simulink model "gm_robot_fis"  (R2023a)
settings: Solver=FixedStepDiscrete  StartTime=0.0  StopTime=10.0  RelTol=1e-3
model workspace (MAT data in the model file):
  x = 1
  y = [100 100 100 100 100 100 100 100 100 100 100 100 ... (256 elements, 256x1)]
libraries: hdlmdlgenlib x75
(part 2 of 3)

== system gm_robot_fis/MATLAB Function ==
  a : Inport  OutDataTypeStr=uint8  PortDimensions=1  SampleTime=0.2
  b : Inport  Port=2  OutDataTypeStr=uint8  PortDimensions=1  SampleTime=0.2
  c : Inport  Port=3  OutDataTypeStr=uint8  PortDimensions=1  SampleTime=0.2
  d : Inport  Port=4  OutDataTypeStr=uint8  PortDimensions=1  SampleTime=0.2
  e : Inport  Port=5  OutDataTypeStr=uint8  PortDimensions=1  SampleTime=0.2
  MATLAB Function : MATLAB Function  TreatAsAtomicUnit=on
  y : Outport  SampleTime=0.2
  wires:
  MATLAB Function/1(y) -> y/1
  a/1 -> MATLAB Function/1(a)
  b/1 -> MATLAB Function/2(b)
  c/1 -> MATLAB Function/3(c)
  d/1 -> MATLAB Function/4(d)
  e/1 -> MATLAB Function/5(e)

== system gm_robot_fis/MinMax Running Resettable ==
  note: Reset
  u : Inport  OutDataTypeStr=uint8  SampleTime=0.2
  R : Inport  Port=2  OutDataTypeStr=uint8  SampleTime=0.2
  Data Type Duplicate : DataTypeDuplicate  DisableCoverage=on  NumInputPorts=3
  MinMax : MinMax  DisableCoverage=on  Inputs=2  OutDataTypeStr=Inherit: Inherit via back propagation  ZeroCross=off
      settings: LockScale=on
  MinMax_out1 : hdlmdlgenlib/Buffer
  Subsystem : Subsystem
  Subsystem_out1 : hdlmdlgenlib/Buffer
  Subsystem_out2 : hdlmdlgenlib/Buffer
  y : Outport  SampleTime=0.2
  wires:
  MinMax_out1/1 -> Data Type Duplicate/1
  Subsystem_out1/1 -> y/1
  Subsystem_out2/1 -> Data Type Duplicate/2
  u/1 -> Data Type Duplicate/3, MinMax/1
  R/1 -> Subsystem/2(R1)
  MinMax/1 -> MinMax_out1/1, Subsystem/1(u1)
  Subsystem/1(y1) -> Subsystem_out1/1
  Subsystem/2(x) -> Subsystem_out2/1, MinMax/2

== system gm_robot_fis/MinMax Running Resettable1 ==
  note: Reset
  u : Inport  OutDataTypeStr=uint8  SampleTime=0.2
  R : Inport  Port=2  OutDataTypeStr=uint8  SampleTime=0.2
  Data Type Duplicate : DataTypeDuplicate  DisableCoverage=on  NumInputPorts=3
  MinMax : MinMax  DisableCoverage=on  Inputs=2  OutDataTypeStr=Inherit: Inherit via back propagation  ZeroCross=off
      settings: LockScale=on
  MinMax_out1 : hdlmdlgenlib/Buffer
  Subsystem : Subsystem
  Subsystem_out1 : hdlmdlgenlib/Buffer
  Subsystem_out2 : hdlmdlgenlib/Buffer
  y : Outport  SampleTime=0.2
  wires:
  MinMax_out1/1 -> Data Type Duplicate/1
  Subsystem_out1/1 -> y/1
  Subsystem_out2/1 -> Data Type Duplicate/2
  u/1 -> Data Type Duplicate/3, MinMax/1
  R/1 -> Subsystem/2(R1)
  MinMax/1 -> MinMax_out1/1, Subsystem/1(u1)
  Subsystem/1(y1) -> Subsystem_out1/1
  Subsystem/2(x) -> Subsystem_out2/1, MinMax/2

== system gm_robot_fis/MinMax Running Resettable10 ==
  note: Reset
  u : Inport  OutDataTypeStr=uint8  SampleTime=0.2
  R : Inport  Port=2  OutDataTypeStr=uint8  SampleTime=0.2
  Data Type Duplicate : DataTypeDuplicate  DisableCoverage=on  NumInputPorts=3
  MinMax : MinMax  DisableCoverage=on  Inputs=2  OutDataTypeStr=Inherit: Inherit via back propagation  ZeroCross=off
      settings: LockScale=on
  MinMax_out1 : hdlmdlgenlib/Buffer
  Subsystem : Subsystem
  Subsystem_out1 : hdlmdlgenlib/Buffer
  Subsystem_out2 : hdlmdlgenlib/Buffer
  y : Outport  SampleTime=0.2
  wires:
  MinMax_out1/1 -> Data Type Duplicate/1
  Subsystem_out1/1 -> y/1
  Subsystem_out2/1 -> Data Type Duplicate/2
  u/1 -> Data Type Duplicate/3, MinMax/1
  R/1 -> Subsystem/2(R1)
  MinMax/1 -> MinMax_out1/1, Subsystem/1(u1)
  Subsystem/1(y1) -> Subsystem_out1/1
  Subsystem/2(x) -> Subsystem_out2/1, MinMax/2

== system gm_robot_fis/MinMax Running Resettable11 ==
  note: Reset
  u : Inport  OutDataTypeStr=uint8  SampleTime=0.2
  R : Inport  Port=2  OutDataTypeStr=uint8  SampleTime=0.2
  Data Type Duplicate : DataTypeDuplicate  DisableCoverage=on  NumInputPorts=3
  MinMax : MinMax  DisableCoverage=on  Inputs=2  OutDataTypeStr=Inherit: Inherit via back propagation  ZeroCross=off
      settings: LockScale=on
  MinMax_out1 : hdlmdlgenlib/Buffer
  Subsystem : Subsystem
  Subsystem_out1 : hdlmdlgenlib/Buffer
  Subsystem_out2 : hdlmdlgenlib/Buffer
  y : Outport  SampleTime=0.2
  wires:
  MinMax_out1/1 -> Data Type Duplicate/1
  Subsystem_out1/1 -> y/1
  Subsystem_out2/1 -> Data Type Duplicate/2
  u/1 -> Data Type Duplicate/3, MinMax/1
  R/1 -> Subsystem/2(R1)
  MinMax/1 -> MinMax_out1/1, Subsystem/1(u1)
  Subsystem/1(y1) -> Subsystem_out1/1
  Subsystem/2(x) -> Subsystem_out2/1, MinMax/2

== system gm_robot_fis/MinMax Running Resettable12 ==
  note: Reset
  u : Inport  OutDataTypeStr=uint8  SampleTime=0.2
  R : Inport  Port=2  OutDataTypeStr=uint8  SampleTime=0.2
  Data Type Duplicate : DataTypeDuplicate  DisableCoverage=on  NumInputPorts=3
  MinMax : MinMax  DisableCoverage=on  Inputs=2  OutDataTypeStr=Inherit: Inherit via back propagation  ZeroCross=off
      settings: LockScale=on
  MinMax_out1 : hdlmdlgenlib/Buffer
  Subsystem : Subsystem
  Subsystem_out1 : hdlmdlgenlib/Buffer
  Subsystem_out2 : hdlmdlgenlib/Buffer
  y : Outport  SampleTime=0.2
  wires:
  MinMax_out1/1 -> Data Type Duplicate/1
  Subsystem_out1/1 -> y/1
  Subsystem_out2/1 -> Data Type Duplicate/2
  u/1 -> Data Type Duplicate/3, MinMax/1
  R/1 -> Subsystem/2(R1)
  MinMax/1 -> MinMax_out1/1, Subsystem/1(u1)
  Subsystem/1(y1) -> Subsystem_out1/1
  Subsystem/2(x) -> Subsystem_out2/1, MinMax/2

== system gm_robot_fis/MinMax Running Resettable13 ==
  note: Reset
  u : Inport  OutDataTypeStr=uint8  SampleTime=0.2
  R : Inport  Port=2  OutDataTypeStr=uint8  SampleTime=0.2
  Data Type Duplicate : DataTypeDuplicate  DisableCoverage=on  NumInputPorts=3
  MinMax : MinMax  DisableCoverage=on  Inputs=2  OutDataTypeStr=Inherit: Inherit via back propagation  ZeroCross=off
      settings: LockScale=on
  MinMax_out1 : hdlmdlgenlib/Buffer
  Subsystem : Subsystem
  Subsystem_out1 : hdlmdlgenlib/Buffer
  Subsystem_out2 : hdlmdlgenlib/Buffer
  y : Outport  SampleTime=0.2
  wires:
  MinMax_out1/1 -> Data Type Duplicate/1
  Subsystem_out1/1 -> y/1
  Subsystem_out2/1 -> Data Type Duplicate/2
  u/1 -> Data Type Duplicate/3, MinMax/1
  R/1 -> Subsystem/2(R1)
  MinMax/1 -> MinMax_out1/1, Subsystem/1(u1)
  Subsystem/1(y1) -> Subsystem_out1/1
  Subsystem/2(x) -> Subsystem_out2/1, MinMax/2

== system gm_robot_fis/MinMax Running Resettable14 ==
  note: Reset
  u : Inport  OutDataTypeStr=uint8  SampleTime=0.2
  R : Inport  Port=2  OutDataTypeStr=uint8  SampleTime=0.2
  Data Type Duplicate : DataTypeDuplicate  DisableCoverage=on  NumInputPorts=3
  MinMax : MinMax  DisableCoverage=on  Inputs=2  OutDataTypeStr=Inherit: Inherit via back propagation  ZeroCross=off
      settings: LockScale=on
  MinMax_out1 : hdlmdlgenlib/Buffer
  Subsystem : Subsystem
  Subsystem_out1 : hdlmdlgenlib/Buffer
  Subsystem_out2 : hdlmdlgenlib/Buffer
  y : Outport  SampleTime=0.2
  wires:
  MinMax_out1/1 -> Data Type Duplicate/1
  Subsystem_out1/1 -> y/1
  Subsystem_out2/1 -> Data Type Duplicate/2
  u/1 -> Data Type Duplicate/3, MinMax/1
  R/1 -> Subsystem/2(R1)
  MinMax/1 -> MinMax_out1/1, Subsystem/1(u1)
  Subsystem/1(y1) -> Subsystem_out1/1
  Subsystem/2(x) -> Subsystem_out2/1, MinMax/2

== system gm_robot_fis/MinMax Running Resettable15 ==
  note: Reset
  u : Inport  OutDataTypeStr=uint8  SampleTime=0.2
  R : Inport  Port=2  OutDataTypeStr=uint8  SampleTime=0.2
  Data Type Duplicate : DataTypeDuplicate  DisableCoverage=on  NumInputPorts=3
  MinMax : MinMax  DisableCoverage=on  Inputs=2  OutDataTypeStr=Inherit: Inherit via back propagation  ZeroCross=off
      settings: LockScale=on
  MinMax_out1 : hdlmdlgenlib/Buffer
  Subsystem : Subsystem
  Subsystem_out1 : hdlmdlgenlib/Buffer
  Subsystem_out2 : hdlmdlgenlib/Buffer
  y : Outport  SampleTime=0.2
  wires:
  MinMax_out1/1 -> Data Type Duplicate/1
  Subsystem_out1/1 -> y/1
  Subsystem_out2/1 -> Data Type Duplicate/2
  u/1 -> Data Type Duplicate/3, MinMax/1
  R/1 -> Subsystem/2(R1)
  MinMax/1 -> MinMax_out1/1, Subsystem/1(u1)
  Subsystem/1(y1) -> Subsystem_out1/1
  Subsystem/2(x) -> Subsystem_out2/1, MinMax/2

== system gm_robot_fis/MinMax Running Resettable16 ==
  note: Reset
  u : Inport  OutDataTypeStr=uint8  SampleTime=0.2
  R : Inport  Port=2  OutDataTypeStr=uint8  SampleTime=0.2
  Data Type Duplicate : DataTypeDuplicate  DisableCoverage=on  NumInputPorts=3
  MinMax : MinMax  DisableCoverage=on  Inputs=2  OutDataTypeStr=Inherit: Inherit via back propagation  ZeroCross=off
      settings: LockScale=on
  MinMax_out1 : hdlmdlgenlib/Buffer
  Subsystem : Subsystem
  Subsystem_out1 : hdlmdlgenlib/Buffer
  Subsystem_out2 : hdlmdlgenlib/Buffer
  y : Outport  SampleTime=0.2
  wires:
  MinMax_out1/1 -> Data Type Duplicate/1
  Subsystem_out1/1 -> y/1
  Subsystem_out2/1 -> Data Type Duplicate/2
  u/1 -> Data Type Duplicate/3, MinMax/1
  R/1 -> Subsystem/2(R1)
  MinMax/1 -> MinMax_out1/1, Subsystem/1(u1)
  Subsystem/1(y1) -> Subsystem_out1/1
  Subsystem/2(x) -> Subsystem_out2/1, MinMax/2

== system gm_robot_fis/MinMax Running Resettable17 ==
  note: Reset
  u : Inport  OutDataTypeStr=uint8  SampleTime=0.2
  R : Inport  Port=2  OutDataTypeStr=uint8  SampleTime=0.2
  Data Type Duplicate : DataTypeDuplicate  DisableCoverage=on  NumInputPorts=3
  MinMax : MinMax  DisableCoverage=on  Inputs=2  OutDataTypeStr=Inherit: Inherit via back propagation  ZeroCross=off
      settings: LockScale=on
  MinMax_out1 : hdlmdlgenlib/Buffer
  Subsystem : Subsystem
  Subsystem_out1 : hdlmdlgenlib/Buffer
  Subsystem_out2 : hdlmdlgenlib/Buffer
  y : Outport  SampleTime=0.2
  wires:
  MinMax_out1/1 -> Data Type Duplicate/1
  Subsystem_out1/1 -> y/1
  Subsystem_out2/1 -> Data Type Duplicate/2
  u/1 -> Data Type Duplicate/3, MinMax/1
  R/1 -> Subsystem/2(R1)
  MinMax/1 -> MinMax_out1/1, Subsystem/1(u1)
  Subsystem/1(y1) -> Subsystem_out1/1
  Subsystem/2(x) -> Subsystem_out2/1, MinMax/2

== system gm_robot_fis/MinMax Running Resettable18 ==
  note: Reset
  u : Inport  OutDataTypeStr=uint8  SampleTime=0.2
  R : Inport  Port=2  OutDataTypeStr=uint8  SampleTime=0.2
  Data Type Duplicate : DataTypeDuplicate  DisableCoverage=on  NumInputPorts=3
  MinMax : MinMax  DisableCoverage=on  Inputs=2  OutDataTypeStr=Inherit: Inherit via back propagation  ZeroCross=off
      settings: LockScale=on
  MinMax_out1 : hdlmdlgenlib/Buffer
  Subsystem : Subsystem
  Subsystem_out1 : hdlmdlgenlib/Buffer
  Subsystem_out2 : hdlmdlgenlib/Buffer
  y : Outport  SampleTime=0.2
  wires:
  MinMax_out1/1 -> Data Type Duplicate/1
  Subsystem_out1/1 -> y/1
  Subsystem_out2/1 -> Data Type Duplicate/2
  u/1 -> Data Type Duplicate/3, MinMax/1
  R/1 -> Subsystem/2(R1)
  MinMax/1 -> MinMax_out1/1, Subsystem/1(u1)
  Subsystem/1(y1) -> Subsystem_out1/1
  Subsystem/2(x) -> Subsystem_out2/1, MinMax/2

== system gm_robot_fis/MinMax Running Resettable19 ==
  note: Reset
  u : Inport  OutDataTypeStr=uint8  SampleTime=0.2
  R : Inport  Port=2  OutDataTypeStr=uint8  SampleTime=0.2
  Data Type Duplicate : DataTypeDuplicate  DisableCoverage=on  NumInputPorts=3
  MinMax : MinMax  DisableCoverage=on  Inputs=2  OutDataTypeStr=Inherit: Inherit via back propagation  ZeroCross=off
      settings: LockScale=on
  MinMax_out1 : hdlmdlgenlib/Buffer
  Subsystem : Subsystem
  Subsystem_out1 : hdlmdlgenlib/Buffer
  Subsystem_out2 : hdlmdlgenlib/Buffer
  y : Outport  SampleTime=0.2
  wires:
  MinMax_out1/1 -> Data Type Duplicate/1
  Subsystem_out1/1 -> y/1
  Subsystem_out2/1 -> Data Type Duplicate/2
  u/1 -> Data Type Duplicate/3, MinMax/1
  R/1 -> Subsystem/2(R1)
  MinMax/1 -> MinMax_out1/1, Subsystem/1(u1)
  Subsystem/1(y1) -> Subsystem_out1/1
  Subsystem/2(x) -> Subsystem_out2/1, MinMax/2

== system gm_robot_fis/MinMax Running Resettable20 ==
  note: Reset
  u : Inport  OutDataTypeStr=uint8  SampleTime=0.2
  R : Inport  Port=2  OutDataTypeStr=uint8  SampleTime=0.2
  Data Type Duplicate : DataTypeDuplicate  DisableCoverage=on  NumInputPorts=3
  MinMax : MinMax  DisableCoverage=on  Inputs=2  OutDataTypeStr=Inherit: Inherit via back propagation  ZeroCross=off
      settings: LockScale=on
  MinMax_out1 : hdlmdlgenlib/Buffer
  Subsystem : Subsystem
  Subsystem_out1 : hdlmdlgenlib/Buffer
  Subsystem_out2 : hdlmdlgenlib/Buffer
  y : Outport  SampleTime=0.2
  wires:
  MinMax_out1/1 -> Data Type Duplicate/1
  Subsystem_out1/1 -> y/1
  Subsystem_out2/1 -> Data Type Duplicate/2
  u/1 -> Data Type Duplicate/3, MinMax/1
  R/1 -> Subsystem/2(R1)
  MinMax/1 -> MinMax_out1/1, Subsystem/1(u1)
  Subsystem/1(y1) -> Subsystem_out1/1
  Subsystem/2(x) -> Subsystem_out2/1, MinMax/2

== system gm_robot_fis/MinMax Running Resettable21 ==
  note: Reset
  u : Inport  OutDataTypeStr=uint8  SampleTime=0.2
  R : Inport  Port=2  OutDataTypeStr=uint8  SampleTime=0.2
  Data Type Duplicate : DataTypeDuplicate  DisableCoverage=on  NumInputPorts=3
  MinMax : MinMax  DisableCoverage=on  Inputs=2  OutDataTypeStr=Inherit: Inherit via back propagation  ZeroCross=off
      settings: LockScale=on
  MinMax_out1 : hdlmdlgenlib/Buffer
  Subsystem : Subsystem
  Subsystem_out1 : hdlmdlgenlib/Buffer
  Subsystem_out2 : hdlmdlgenlib/Buffer
  y : Outport  SampleTime=0.2
  wires:
  MinMax_out1/1 -> Data Type Duplicate/1
  Subsystem_out1/1 -> y/1
  Subsystem_out2/1 -> Data Type Duplicate/2
  u/1 -> Data Type Duplicate/3, MinMax/1
  R/1 -> Subsystem/2(R1)
  MinMax/1 -> MinMax_out1/1, Subsystem/1(u1)
  Subsystem/1(y1) -> Subsystem_out1/1
  Subsystem/2(x) -> Subsystem_out2/1, MinMax/2

== system gm_robot_fis/MinMax Running Resettable22 ==
  note: Reset
  u : Inport  OutDataTypeStr=uint8  SampleTime=0.2
  R : Inport  Port=2  OutDataTypeStr=uint8  SampleTime=0.2
  Data Type Duplicate : DataTypeDuplicate  DisableCoverage=on  NumInputPorts=3
  MinMax : MinMax  DisableCoverage=on  Inputs=2  OutDataTypeStr=Inherit: Inherit via back propagation  ZeroCross=off
      settings: LockScale=on
  MinMax_out1 : hdlmdlgenlib/Buffer
  Subsystem : Subsystem
  Subsystem_out1 : hdlmdlgenlib/Buffer
  Subsystem_out2 : hdlmdlgenlib/Buffer
  y : Outport  SampleTime=0.2
  wires:
  MinMax_out1/1 -> Data Type Duplicate/1
  Subsystem_out1/1 -> y/1
  Subsystem_out2/1 -> Data Type Duplicate/2
  u/1 -> Data Type Duplicate/3, MinMax/1
  R/1 -> Subsystem/2(R1)
  MinMax/1 -> MinMax_out1/1, Subsystem/1(u1)
  Subsystem/1(y1) -> Subsystem_out1/1
  Subsystem/2(x) -> Subsystem_out2/1, MinMax/2

== system gm_robot_fis/MinMax Running Resettable23 ==
  note: Reset
  u : Inport  OutDataTypeStr=uint8  SampleTime=0.2
  R : Inport  Port=2  OutDataTypeStr=uint8  SampleTime=0.2
  Data Type Duplicate : DataTypeDuplicate  DisableCoverage=on  NumInputPorts=3
  MinMax : MinMax  DisableCoverage=on  Inputs=2  OutDataTypeStr=Inherit: Inherit via back propagation  ZeroCross=off
      settings: LockScale=on
  MinMax_out1 : hdlmdlgenlib/Buffer
  Subsystem : Subsystem
  Subsystem_out1 : hdlmdlgenlib/Buffer
  Subsystem_out2 : hdlmdlgenlib/Buffer
  y : Outport  SampleTime=0.2
  wires:
  MinMax_out1/1 -> Data Type Duplicate/1
  Subsystem_out1/1 -> y/1
  Subsystem_out2/1 -> Data Type Duplicate/2
  u/1 -> Data Type Duplicate/3, MinMax/1
  R/1 -> Subsystem/2(R1)
  MinMax/1 -> MinMax_out1/1, Subsystem/1(u1)
  Subsystem/1(y1) -> Subsystem_out1/1
  Subsystem/2(x) -> Subsystem_out2/1, MinMax/2

== system gm_robot_fis/MinMax Running Resettable24 ==
  note: Reset
  u : Inport  OutDataTypeStr=uint8  SampleTime=0.2
  R : Inport  Port=2  OutDataTypeStr=uint8  SampleTime=0.2
  Data Type Duplicate : DataTypeDuplicate  DisableCoverage=on  NumInputPorts=3
  MinMax : MinMax  DisableCoverage=on  Inputs=2  OutDataTypeStr=Inherit: Inherit via back propagation  ZeroCross=off
      settings: LockScale=on
  MinMax_out1 : hdlmdlgenlib/Buffer
  Subsystem : Subsystem
  Subsystem_out1 : hdlmdlgenlib/Buffer
  Subsystem_out2 : hdlmdlgenlib/Buffer
  y : Outport  SampleTime=0.2
  wires:
  MinMax_out1/1 -> Data Type Duplicate/1
  Subsystem_out1/1 -> y/1
  Subsystem_out2/1 -> Data Type Duplicate/2
  u/1 -> Data Type Duplicate/3, MinMax/1
  R/1 -> Subsystem/2(R1)
  MinMax/1 -> MinMax_out1/1, Subsystem/1(u1)
  Subsystem/1(y1) -> Subsystem_out1/1
  Subsystem/2(x) -> Subsystem_out2/1, MinMax/2

== system gm_robot_fis/MinMax Running Resettable25 ==
  note: Reset
  u : Inport  OutDataTypeStr=uint8  SampleTime=0.2
  R : Inport  Port=2  OutDataTypeStr=uint8  SampleTime=0.2
  Data Type Duplicate : DataTypeDuplicate  DisableCoverage=on  NumInputPorts=3
  MinMax : MinMax  DisableCoverage=on  Inputs=2  OutDataTypeStr=Inherit: Inherit via back propagation  ZeroCross=off
      settings: LockScale=on
  MinMax_out1 : hdlmdlgenlib/Buffer
  Subsystem : Subsystem
  Subsystem_out1 : hdlmdlgenlib/Buffer
  Subsystem_out2 : hdlmdlgenlib/Buffer
  y : Outport  SampleTime=0.2
  wires:
  MinMax_out1/1 -> Data Type Duplicate/1
  Subsystem_out1/1 -> y/1
  Subsystem_out2/1 -> Data Type Duplicate/2
  u/1 -> Data Type Duplicate/3, MinMax/1
  R/1 -> Subsystem/2(R1)
  MinMax/1 -> MinMax_out1/1, Subsystem/1(u1)
  Subsystem/1(y1) -> Subsystem_out1/1
  Subsystem/2(x) -> Subsystem_out2/1, MinMax/2

== system gm_robot_fis/MinMax Running Resettable3 ==
  note: Reset
  u : Inport  OutDataTypeStr=uint8  SampleTime=0.2
  R : Inport  Port=2  OutDataTypeStr=uint8  SampleTime=0.2
  Data Type Duplicate : DataTypeDuplicate  DisableCoverage=on  NumInputPorts=3
  MinMax : MinMax  DisableCoverage=on  Inputs=2  OutDataTypeStr=Inherit: Inherit via back propagation  ZeroCross=off
      settings: LockScale=on
  MinMax_out1 : hdlmdlgenlib/Buffer
  Subsystem : Subsystem
  Subsystem_out1 : hdlmdlgenlib/Buffer
  Subsystem_out2 : hdlmdlgenlib/Buffer
  y : Outport  SampleTime=0.2
  wires:
  MinMax_out1/1 -> Data Type Duplicate/1
  Subsystem_out1/1 -> y/1
  Subsystem_out2/1 -> Data Type Duplicate/2
  u/1 -> Data Type Duplicate/3, MinMax/1
  R/1 -> Subsystem/2(R1)
  MinMax/1 -> MinMax_out1/1, Subsystem/1(u1)
  Subsystem/1(y1) -> Subsystem_out1/1
  Subsystem/2(x) -> Subsystem_out2/1, MinMax/2

== system gm_robot_fis/MinMax Running Resettable4 ==
  note: Reset
  u : Inport  OutDataTypeStr=uint8  SampleTime=0.2
  R : Inport  Port=2  OutDataTypeStr=uint8  SampleTime=0.2
  Data Type Duplicate : DataTypeDuplicate  DisableCoverage=on  NumInputPorts=3
  MinMax : MinMax  DisableCoverage=on  Inputs=2  OutDataTypeStr=Inherit: Inherit via back propagation  ZeroCross=off
      settings: LockScale=on
  MinMax_out1 : hdlmdlgenlib/Buffer
  Subsystem : Subsystem
  Subsystem_out1 : hdlmdlgenlib/Buffer
  Subsystem_out2 : hdlmdlgenlib/Buffer
  y : Outport  SampleTime=0.2
  wires:
  MinMax_out1/1 -> Data Type Duplicate/1
  Subsystem_out1/1 -> y/1
  Subsystem_out2/1 -> Data Type Duplicate/2
  u/1 -> Data Type Duplicate/3, MinMax/1
  R/1 -> Subsystem/2(R1)
  MinMax/1 -> MinMax_out1/1, Subsystem/1(u1)
  Subsystem/1(y1) -> Subsystem_out1/1
  Subsystem/2(x) -> Subsystem_out2/1, MinMax/2

== system gm_robot_fis/MinMax Running Resettable5 ==
  note: Reset
  u : Inport  OutDataTypeStr=uint8  SampleTime=0.2
  R : Inport  Port=2  OutDataTypeStr=uint8  SampleTime=0.2
  Data Type Duplicate : DataTypeDuplicate  DisableCoverage=on  NumInputPorts=3
  MinMax : MinMax  DisableCoverage=on  Inputs=2  OutDataTypeStr=Inherit: Inherit via back propagation  ZeroCross=off
      settings: LockScale=on
  MinMax_out1 : hdlmdlgenlib/Buffer
  Subsystem : Subsystem
  Subsystem_out1 : hdlmdlgenlib/Buffer
  Subsystem_out2 : hdlmdlgenlib/Buffer
  y : Outport  SampleTime=0.2
  wires:
  MinMax_out1/1 -> Data Type Duplicate/1
  Subsystem_out1/1 -> y/1
  Subsystem_out2/1 -> Data Type Duplicate/2
  u/1 -> Data Type Duplicate/3, MinMax/1
  R/1 -> Subsystem/2(R1)
  MinMax/1 -> MinMax_out1/1, Subsystem/1(u1)
  Subsystem/1(y1) -> Subsystem_out1/1
  Subsystem/2(x) -> Subsystem_out2/1, MinMax/2

== system gm_robot_fis/MinMax Running Resettable6 ==
  note: Reset
  u : Inport  OutDataTypeStr=uint8  SampleTime=0.2
  R : Inport  Port=2  OutDataTypeStr=uint8  SampleTime=0.2
  Data Type Duplicate : DataTypeDuplicate  DisableCoverage=on  NumInputPorts=3
  MinMax : MinMax  DisableCoverage=on  Inputs=2  OutDataTypeStr=Inherit: Inherit via back propagation  ZeroCross=off
      settings: LockScale=on
  MinMax_out1 : hdlmdlgenlib/Buffer
  Subsystem : Subsystem
  Subsystem_out1 : hdlmdlgenlib/Buffer
  Subsystem_out2 : hdlmdlgenlib/Buffer
  y : Outport  SampleTime=0.2
  wires:
  MinMax_out1/1 -> Data Type Duplicate/1
  Subsystem_out1/1 -> y/1
  Subsystem_out2/1 -> Data Type Duplicate/2
  u/1 -> Data Type Duplicate/3, MinMax/1
  R/1 -> Subsystem/2(R1)
  MinMax/1 -> MinMax_out1/1, Subsystem/1(u1)
  Subsystem/1(y1) -> Subsystem_out1/1
  Subsystem/2(x) -> Subsystem_out2/1, MinMax/2

== system gm_robot_fis/MinMax Running Resettable7 ==
  note: Reset
  u : Inport  OutDataTypeStr=uint8  SampleTime=0.2
  R : Inport  Port=2  OutDataTypeStr=uint8  SampleTime=0.2
  Data Type Duplicate : DataTypeDuplicate  DisableCoverage=on  NumInputPorts=3
  MinMax : MinMax  DisableCoverage=on  Inputs=2  OutDataTypeStr=Inherit: Inherit via back propagation  ZeroCross=off
      settings: LockScale=on
  MinMax_out1 : hdlmdlgenlib/Buffer
  Subsystem : Subsystem
  Subsystem_out1 : hdlmdlgenlib/Buffer
  Subsystem_out2 : hdlmdlgenlib/Buffer
  y : Outport  SampleTime=0.2
  wires:
  MinMax_out1/1 -> Data Type Duplicate/1
  Subsystem_out1/1 -> y/1
  Subsystem_out2/1 -> Data Type Duplicate/2
  u/1 -> Data Type Duplicate/3, MinMax/1
  R/1 -> Subsystem/2(R1)
  MinMax/1 -> MinMax_out1/1, Subsystem/1(u1)
  Subsystem/1(y1) -> Subsystem_out1/1
  Subsystem/2(x) -> Subsystem_out2/1, MinMax/2

== system gm_robot_fis/MinMax Running Resettable8 ==
  note: Reset
  u : Inport  OutDataTypeStr=uint8  SampleTime=0.2
  R : Inport  Port=2  OutDataTypeStr=uint8  SampleTime=0.2
  Data Type Duplicate : DataTypeDuplicate  DisableCoverage=on  NumInputPorts=3
  MinMax : MinMax  DisableCoverage=on  Inputs=2  OutDataTypeStr=Inherit: Inherit via back propagation  ZeroCross=off
      settings: LockScale=on
  MinMax_out1 : hdlmdlgenlib/Buffer
  Subsystem : Subsystem
  Subsystem_out1 : hdlmdlgenlib/Buffer
  Subsystem_out2 : hdlmdlgenlib/Buffer
  y : Outport  SampleTime=0.2
  wires:
  MinMax_out1/1 -> Data Type Duplicate/1
  Subsystem_out1/1 -> y/1
  Subsystem_out2/1 -> Data Type Duplicate/2
  u/1 -> Data Type Duplicate/3, MinMax/1
  R/1 -> Subsystem/2(R1)
  MinMax/1 -> MinMax_out1/1, Subsystem/1(u1)
  Subsystem/1(y1) -> Subsystem_out1/1
  Subsystem/2(x) -> Subsystem_out2/1, MinMax/2

== system gm_robot_fis/MinMax Running Resettable9 ==
  note: Reset
  u : Inport  OutDataTypeStr=uint8  SampleTime=0.2
  R : Inport  Port=2  OutDataTypeStr=uint8  SampleTime=0.2
  Data Type Duplicate : DataTypeDuplicate  DisableCoverage=on  NumInputPorts=3
  MinMax : MinMax  DisableCoverage=on  Inputs=2  OutDataTypeStr=Inherit: Inherit via back propagation  ZeroCross=off
      settings: LockScale=on
  MinMax_out1 : hdlmdlgenlib/Buffer
  Subsystem : Subsystem
  Subsystem_out1 : hdlmdlgenlib/Buffer
  Subsystem_out2 : hdlmdlgenlib/Buffer
  y : Outport  SampleTime=0.2
  wires:
  MinMax_out1/1 -> Data Type Duplicate/1
  Subsystem_out1/1 -> y/1
  Subsystem_out2/1 -> Data Type Duplicate/2
  u/1 -> Data Type Duplicate/3, MinMax/1
  R/1 -> Subsystem/2(R1)
  MinMax/1 -> MinMax_out1/1, Subsystem/1(u1)
  Subsystem/1(y1) -> Subsystem_out1/1
  Subsystem/2(x) -> Subsystem_out2/1, MinMax/2

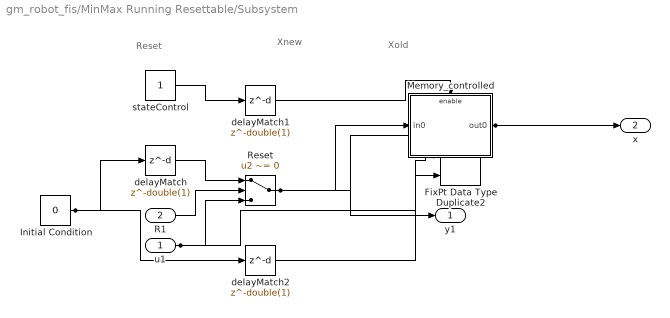
== system gm_robot_fis/MinMax Running Resettable/Subsystem ==
  note: Reset
  note: Xnew
  note: Xold
  u1 : Inport  OutDataTypeStr=uint8  PortDimensions=1  SampleTime=0.2
  R1 : Inport  Port=2  OutDataTypeStr=uint8  PortDimensions=1  SampleTime=0.2
  FixPt Data Type Duplicate2 : DataTypeDuplicate  DisableCoverage=on  NumInputPorts=4
  Initial Condition : Constant  Value=0  OutDataTypeStr=uint8  SampleTime=0.2
  Memory_controlled : Subsystem
  Reset : Switch  Criteria=u2 ~= 0  Threshold=double(0)  OutDataTypeStr=uint8  SampleTime=0.2  SaturateOnIntegerOverflow=off  InputSameDT=off
  delayMatch : Delay  DelayLength=double(1)  InitialCondition=0  SampleTime=0.2
  delayMatch1 : Delay  DelayLength=double(1)  InitialCondition=0  SampleTime=0.2
  delayMatch2 : Delay  DelayLength=double(1)  InitialCondition=0  SampleTime=0.2
  stateControl : Constant  OutDataTypeStr=boolean  SampleTime=0.2
  y1 : Outport  SampleTime=0.2
  x : Outport  Port=2  SampleTime=0.2
  wires:
  delayMatch/1 -> Reset/1
  Memory_controlled/1(out0) -> FixPt Data Type Duplicate2/1, x/1
  Reset/1 -> Memory_controlled/1(in0), FixPt Data Type Duplicate2/2, y1/1
  delayMatch1/1 -> Memory_controlled/Enable
  u1/1 -> Reset/3, FixPt Data Type Duplicate2/4
  R1/1 -> Reset/2
  delayMatch2/1 -> FixPt Data Type Duplicate2/3
  stateControl/1 -> delayMatch1/1
  Initial Condition/1 -> delayMatch2/1, delayMatch/1

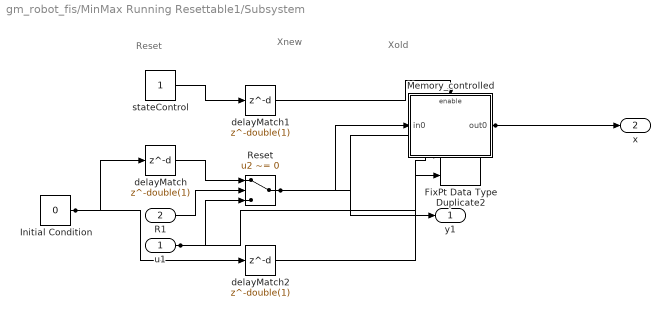
== system gm_robot_fis/MinMax Running Resettable1/Subsystem ==
  note: Reset
  note: Xnew
  note: Xold
  u1 : Inport  OutDataTypeStr=uint8  PortDimensions=1  SampleTime=0.2
  R1 : Inport  Port=2  OutDataTypeStr=uint8  PortDimensions=1  SampleTime=0.2
  FixPt Data Type Duplicate2 : DataTypeDuplicate  DisableCoverage=on  NumInputPorts=4
  Initial Condition : Constant  Value=0  OutDataTypeStr=uint8  SampleTime=0.2
  Memory_controlled : Subsystem
  Reset : Switch  Criteria=u2 ~= 0  Threshold=double(0)  OutDataTypeStr=uint8  SampleTime=0.2  SaturateOnIntegerOverflow=off  InputSameDT=off
  delayMatch : Delay  DelayLength=double(1)  InitialCondition=0  SampleTime=0.2
  delayMatch1 : Delay  DelayLength=double(1)  InitialCondition=0  SampleTime=0.2
  delayMatch2 : Delay  DelayLength=double(1)  InitialCondition=0  SampleTime=0.2
  stateControl : Constant  OutDataTypeStr=boolean  SampleTime=0.2
  y1 : Outport  SampleTime=0.2
  x : Outport  Port=2  SampleTime=0.2
  wires:
  delayMatch/1 -> Reset/1
  Memory_controlled/1(out0) -> FixPt Data Type Duplicate2/1, x/1
  Reset/1 -> Memory_controlled/1(in0), FixPt Data Type Duplicate2/2, y1/1
  delayMatch1/1 -> Memory_controlled/Enable
  u1/1 -> Reset/3, FixPt Data Type Duplicate2/4
  R1/1 -> Reset/2
  delayMatch2/1 -> FixPt Data Type Duplicate2/3
  stateControl/1 -> delayMatch1/1
  Initial Condition/1 -> delayMatch2/1, delayMatch/1

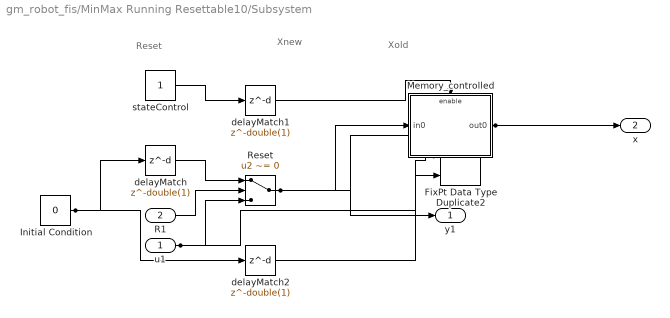
== system gm_robot_fis/MinMax Running Resettable10/Subsystem ==
  note: Reset
  note: Xnew
  note: Xold
  u1 : Inport  OutDataTypeStr=uint8  PortDimensions=1  SampleTime=0.2
  R1 : Inport  Port=2  OutDataTypeStr=uint8  PortDimensions=1  SampleTime=0.2
  FixPt Data Type Duplicate2 : DataTypeDuplicate  DisableCoverage=on  NumInputPorts=4
  Initial Condition : Constant  Value=0  OutDataTypeStr=uint8  SampleTime=0.2
  Memory_controlled : Subsystem
  Reset : Switch  Criteria=u2 ~= 0  Threshold=double(0)  OutDataTypeStr=uint8  SampleTime=0.2  SaturateOnIntegerOverflow=off  InputSameDT=off
  delayMatch : Delay  DelayLength=double(1)  InitialCondition=0  SampleTime=0.2
  delayMatch1 : Delay  DelayLength=double(1)  InitialCondition=0  SampleTime=0.2
  delayMatch2 : Delay  DelayLength=double(1)  InitialCondition=0  SampleTime=0.2
  stateControl : Constant  OutDataTypeStr=boolean  SampleTime=0.2
  y1 : Outport  SampleTime=0.2
  x : Outport  Port=2  SampleTime=0.2
  wires:
  delayMatch/1 -> Reset/1
  Memory_controlled/1(out0) -> FixPt Data Type Duplicate2/1, x/1
  Reset/1 -> Memory_controlled/1(in0), FixPt Data Type Duplicate2/2, y1/1
  delayMatch1/1 -> Memory_controlled/Enable
  u1/1 -> Reset/3, FixPt Data Type Duplicate2/4
  R1/1 -> Reset/2
  delayMatch2/1 -> FixPt Data Type Duplicate2/3
  stateControl/1 -> delayMatch1/1
  Initial Condition/1 -> delayMatch2/1, delayMatch/1

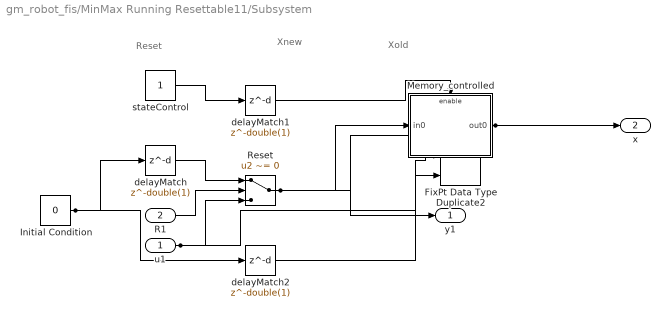
== system gm_robot_fis/MinMax Running Resettable11/Subsystem ==
  note: Reset
  note: Xnew
  note: Xold
  u1 : Inport  OutDataTypeStr=uint8  PortDimensions=1  SampleTime=0.2
  R1 : Inport  Port=2  OutDataTypeStr=uint8  PortDimensions=1  SampleTime=0.2
  FixPt Data Type Duplicate2 : DataTypeDuplicate  DisableCoverage=on  NumInputPorts=4
  Initial Condition : Constant  Value=0  OutDataTypeStr=uint8  SampleTime=0.2
  Memory_controlled : Subsystem
  Reset : Switch  Criteria=u2 ~= 0  Threshold=double(0)  OutDataTypeStr=uint8  SampleTime=0.2  SaturateOnIntegerOverflow=off  InputSameDT=off
  delayMatch : Delay  DelayLength=double(1)  InitialCondition=0  SampleTime=0.2
  delayMatch1 : Delay  DelayLength=double(1)  InitialCondition=0  SampleTime=0.2
  delayMatch2 : Delay  DelayLength=double(1)  InitialCondition=0  SampleTime=0.2
  stateControl : Constant  OutDataTypeStr=boolean  SampleTime=0.2
  y1 : Outport  SampleTime=0.2
  x : Outport  Port=2  SampleTime=0.2
  wires:
  delayMatch/1 -> Reset/1
  Memory_controlled/1(out0) -> FixPt Data Type Duplicate2/1, x/1
  Reset/1 -> Memory_controlled/1(in0), FixPt Data Type Duplicate2/2, y1/1
  delayMatch1/1 -> Memory_controlled/Enable
  u1/1 -> Reset/3, FixPt Data Type Duplicate2/4
  R1/1 -> Reset/2
  delayMatch2/1 -> FixPt Data Type Duplicate2/3
  stateControl/1 -> delayMatch1/1
  Initial Condition/1 -> delayMatch2/1, delayMatch/1

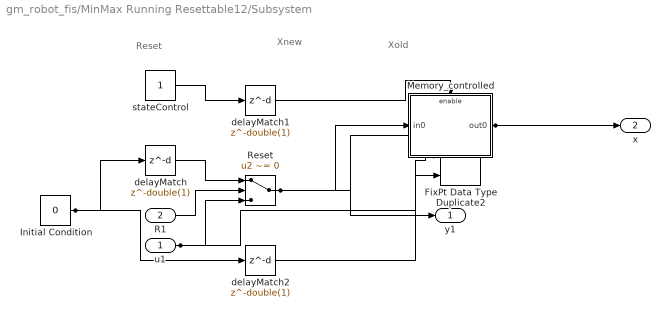
== system gm_robot_fis/MinMax Running Resettable12/Subsystem ==
  note: Reset
  note: Xnew
  note: Xold
  u1 : Inport  OutDataTypeStr=uint8  PortDimensions=1  SampleTime=0.2
  R1 : Inport  Port=2  OutDataTypeStr=uint8  PortDimensions=1  SampleTime=0.2
  FixPt Data Type Duplicate2 : DataTypeDuplicate  DisableCoverage=on  NumInputPorts=4
  Initial Condition : Constant  Value=0  OutDataTypeStr=uint8  SampleTime=0.2
  Memory_controlled : Subsystem
  Reset : Switch  Criteria=u2 ~= 0  Threshold=double(0)  OutDataTypeStr=uint8  SampleTime=0.2  SaturateOnIntegerOverflow=off  InputSameDT=off
  delayMatch : Delay  DelayLength=double(1)  InitialCondition=0  SampleTime=0.2
  delayMatch1 : Delay  DelayLength=double(1)  InitialCondition=0  SampleTime=0.2
  delayMatch2 : Delay  DelayLength=double(1)  InitialCondition=0  SampleTime=0.2
  stateControl : Constant  OutDataTypeStr=boolean  SampleTime=0.2
  y1 : Outport  SampleTime=0.2
  x : Outport  Port=2  SampleTime=0.2
  wires:
  delayMatch/1 -> Reset/1
  Memory_controlled/1(out0) -> FixPt Data Type Duplicate2/1, x/1
  Reset/1 -> Memory_controlled/1(in0), FixPt Data Type Duplicate2/2, y1/1
  delayMatch1/1 -> Memory_controlled/Enable
  u1/1 -> Reset/3, FixPt Data Type Duplicate2/4
  R1/1 -> Reset/2
  delayMatch2/1 -> FixPt Data Type Duplicate2/3
  stateControl/1 -> delayMatch1/1
  Initial Condition/1 -> delayMatch2/1, delayMatch/1

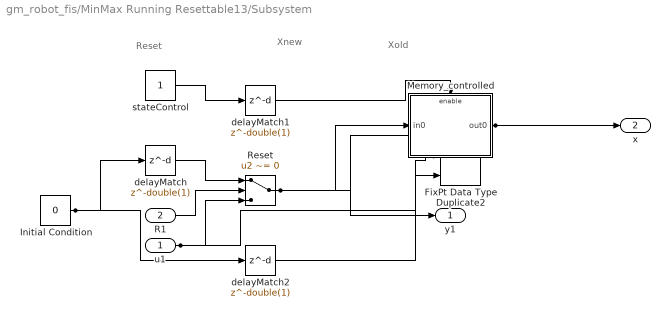
== system gm_robot_fis/MinMax Running Resettable13/Subsystem ==
  note: Reset
  note: Xnew
  note: Xold
  u1 : Inport  OutDataTypeStr=uint8  PortDimensions=1  SampleTime=0.2
  R1 : Inport  Port=2  OutDataTypeStr=uint8  PortDimensions=1  SampleTime=0.2
  FixPt Data Type Duplicate2 : DataTypeDuplicate  DisableCoverage=on  NumInputPorts=4
  Initial Condition : Constant  Value=0  OutDataTypeStr=uint8  SampleTime=0.2
  Memory_controlled : Subsystem
  Reset : Switch  Criteria=u2 ~= 0  Threshold=double(0)  OutDataTypeStr=uint8  SampleTime=0.2  SaturateOnIntegerOverflow=off  InputSameDT=off
  delayMatch : Delay  DelayLength=double(1)  InitialCondition=0  SampleTime=0.2
  delayMatch1 : Delay  DelayLength=double(1)  InitialCondition=0  SampleTime=0.2
  delayMatch2 : Delay  DelayLength=double(1)  InitialCondition=0  SampleTime=0.2
  stateControl : Constant  OutDataTypeStr=boolean  SampleTime=0.2
  y1 : Outport  SampleTime=0.2
  x : Outport  Port=2  SampleTime=0.2
  wires:
  delayMatch/1 -> Reset/1
  Memory_controlled/1(out0) -> FixPt Data Type Duplicate2/1, x/1
  Reset/1 -> Memory_controlled/1(in0), FixPt Data Type Duplicate2/2, y1/1
  delayMatch1/1 -> Memory_controlled/Enable
  u1/1 -> Reset/3, FixPt Data Type Duplicate2/4
  R1/1 -> Reset/2
  delayMatch2/1 -> FixPt Data Type Duplicate2/3
  stateControl/1 -> delayMatch1/1
  Initial Condition/1 -> delayMatch2/1, delayMatch/1

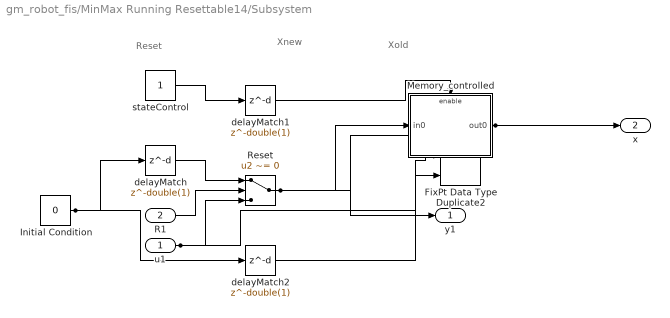
== system gm_robot_fis/MinMax Running Resettable14/Subsystem ==
  note: Reset
  note: Xnew
  note: Xold
  u1 : Inport  OutDataTypeStr=uint8  PortDimensions=1  SampleTime=0.2
  R1 : Inport  Port=2  OutDataTypeStr=uint8  PortDimensions=1  SampleTime=0.2
  FixPt Data Type Duplicate2 : DataTypeDuplicate  DisableCoverage=on  NumInputPorts=4
  Initial Condition : Constant  Value=0  OutDataTypeStr=uint8  SampleTime=0.2
  Memory_controlled : Subsystem
  Reset : Switch  Criteria=u2 ~= 0  Threshold=double(0)  OutDataTypeStr=uint8  SampleTime=0.2  SaturateOnIntegerOverflow=off  InputSameDT=off
  delayMatch : Delay  DelayLength=double(1)  InitialCondition=0  SampleTime=0.2
  delayMatch1 : Delay  DelayLength=double(1)  InitialCondition=0  SampleTime=0.2
  delayMatch2 : Delay  DelayLength=double(1)  InitialCondition=0  SampleTime=0.2
  stateControl : Constant  OutDataTypeStr=boolean  SampleTime=0.2
  y1 : Outport  SampleTime=0.2
  x : Outport  Port=2  SampleTime=0.2
  wires:
  delayMatch/1 -> Reset/1
  Memory_controlled/1(out0) -> FixPt Data Type Duplicate2/1, x/1
  Reset/1 -> Memory_controlled/1(in0), FixPt Data Type Duplicate2/2, y1/1
  delayMatch1/1 -> Memory_controlled/Enable
  u1/1 -> Reset/3, FixPt Data Type Duplicate2/4
  R1/1 -> Reset/2
  delayMatch2/1 -> FixPt Data Type Duplicate2/3
  stateControl/1 -> delayMatch1/1
  Initial Condition/1 -> delayMatch2/1, delayMatch/1

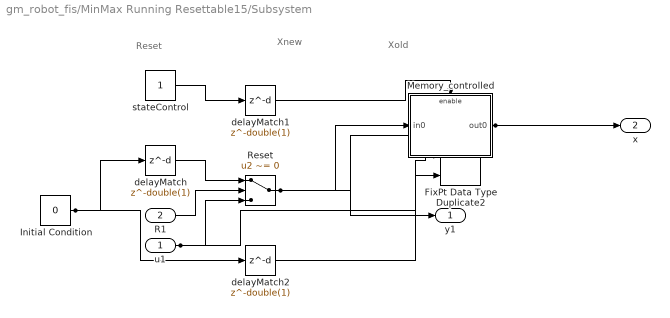
== system gm_robot_fis/MinMax Running Resettable15/Subsystem ==
  note: Reset
  note: Xnew
  note: Xold
  u1 : Inport  OutDataTypeStr=uint8  PortDimensions=1  SampleTime=0.2
  R1 : Inport  Port=2  OutDataTypeStr=uint8  PortDimensions=1  SampleTime=0.2
  FixPt Data Type Duplicate2 : DataTypeDuplicate  DisableCoverage=on  NumInputPorts=4
  Initial Condition : Constant  Value=0  OutDataTypeStr=uint8  SampleTime=0.2
  Memory_controlled : Subsystem
  Reset : Switch  Criteria=u2 ~= 0  Threshold=double(0)  OutDataTypeStr=uint8  SampleTime=0.2  SaturateOnIntegerOverflow=off  InputSameDT=off
  delayMatch : Delay  DelayLength=double(1)  InitialCondition=0  SampleTime=0.2
  delayMatch1 : Delay  DelayLength=double(1)  InitialCondition=0  SampleTime=0.2
  delayMatch2 : Delay  DelayLength=double(1)  InitialCondition=0  SampleTime=0.2
  stateControl : Constant  OutDataTypeStr=boolean  SampleTime=0.2
  y1 : Outport  SampleTime=0.2
  x : Outport  Port=2  SampleTime=0.2
  wires:
  delayMatch/1 -> Reset/1
  Memory_controlled/1(out0) -> FixPt Data Type Duplicate2/1, x/1
  Reset/1 -> Memory_controlled/1(in0), FixPt Data Type Duplicate2/2, y1/1
  delayMatch1/1 -> Memory_controlled/Enable
  u1/1 -> Reset/3, FixPt Data Type Duplicate2/4
  R1/1 -> Reset/2
  delayMatch2/1 -> FixPt Data Type Duplicate2/3
  stateControl/1 -> delayMatch1/1
  Initial Condition/1 -> delayMatch2/1, delayMatch/1

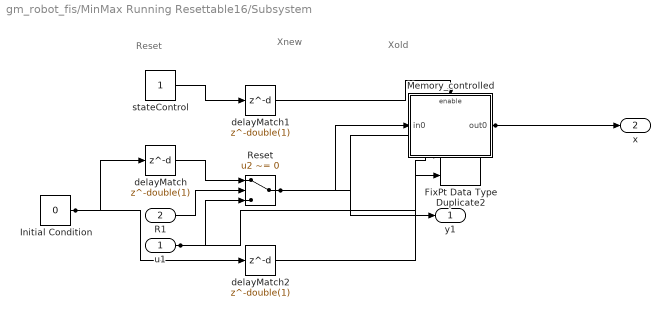
== system gm_robot_fis/MinMax Running Resettable16/Subsystem ==
  note: Reset
  note: Xnew
  note: Xold
  u1 : Inport  OutDataTypeStr=uint8  PortDimensions=1  SampleTime=0.2
  R1 : Inport  Port=2  OutDataTypeStr=uint8  PortDimensions=1  SampleTime=0.2
  FixPt Data Type Duplicate2 : DataTypeDuplicate  DisableCoverage=on  NumInputPorts=4
  Initial Condition : Constant  Value=0  OutDataTypeStr=uint8  SampleTime=0.2
  Memory_controlled : Subsystem
  Reset : Switch  Criteria=u2 ~= 0  Threshold=double(0)  OutDataTypeStr=uint8  SampleTime=0.2  SaturateOnIntegerOverflow=off  InputSameDT=off
  delayMatch : Delay  DelayLength=double(1)  InitialCondition=0  SampleTime=0.2
  delayMatch1 : Delay  DelayLength=double(1)  InitialCondition=0  SampleTime=0.2
  delayMatch2 : Delay  DelayLength=double(1)  InitialCondition=0  SampleTime=0.2
  stateControl : Constant  OutDataTypeStr=boolean  SampleTime=0.2
  y1 : Outport  SampleTime=0.2
  x : Outport  Port=2  SampleTime=0.2
  wires:
  delayMatch/1 -> Reset/1
  Memory_controlled/1(out0) -> FixPt Data Type Duplicate2/1, x/1
  Reset/1 -> Memory_controlled/1(in0), FixPt Data Type Duplicate2/2, y1/1
  delayMatch1/1 -> Memory_controlled/Enable
  u1/1 -> Reset/3, FixPt Data Type Duplicate2/4
  R1/1 -> Reset/2
  delayMatch2/1 -> FixPt Data Type Duplicate2/3
  stateControl/1 -> delayMatch1/1
  Initial Condition/1 -> delayMatch2/1, delayMatch/1

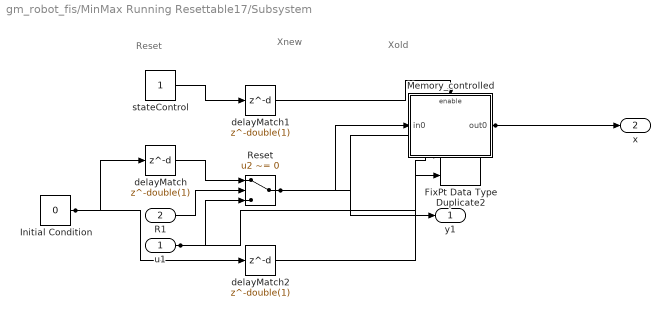
== system gm_robot_fis/MinMax Running Resettable17/Subsystem ==
  note: Reset
  note: Xnew
  note: Xold
  u1 : Inport  OutDataTypeStr=uint8  PortDimensions=1  SampleTime=0.2
  R1 : Inport  Port=2  OutDataTypeStr=uint8  PortDimensions=1  SampleTime=0.2
  FixPt Data Type Duplicate2 : DataTypeDuplicate  DisableCoverage=on  NumInputPorts=4
  Initial Condition : Constant  Value=0  OutDataTypeStr=uint8  SampleTime=0.2
  Memory_controlled : Subsystem
  Reset : Switch  Criteria=u2 ~= 0  Threshold=double(0)  OutDataTypeStr=uint8  SampleTime=0.2  SaturateOnIntegerOverflow=off  InputSameDT=off
  delayMatch : Delay  DelayLength=double(1)  InitialCondition=0  SampleTime=0.2
  delayMatch1 : Delay  DelayLength=double(1)  InitialCondition=0  SampleTime=0.2
  delayMatch2 : Delay  DelayLength=double(1)  InitialCondition=0  SampleTime=0.2
  stateControl : Constant  OutDataTypeStr=boolean  SampleTime=0.2
  y1 : Outport  SampleTime=0.2
  x : Outport  Port=2  SampleTime=0.2
  wires:
  delayMatch/1 -> Reset/1
  Memory_controlled/1(out0) -> FixPt Data Type Duplicate2/1, x/1
  Reset/1 -> Memory_controlled/1(in0), FixPt Data Type Duplicate2/2, y1/1
  delayMatch1/1 -> Memory_controlled/Enable
  u1/1 -> Reset/3, FixPt Data Type Duplicate2/4
  R1/1 -> Reset/2
  delayMatch2/1 -> FixPt Data Type Duplicate2/3
  stateControl/1 -> delayMatch1/1
  Initial Condition/1 -> delayMatch2/1, delayMatch/1

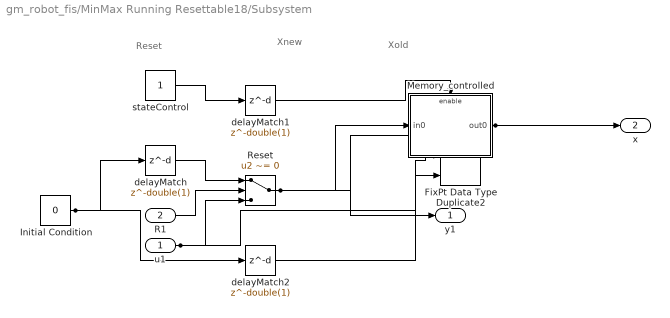
== system gm_robot_fis/MinMax Running Resettable18/Subsystem ==
  note: Reset
  note: Xnew
  note: Xold
  u1 : Inport  OutDataTypeStr=uint8  PortDimensions=1  SampleTime=0.2
  R1 : Inport  Port=2  OutDataTypeStr=uint8  PortDimensions=1  SampleTime=0.2
  FixPt Data Type Duplicate2 : DataTypeDuplicate  DisableCoverage=on  NumInputPorts=4
  Initial Condition : Constant  Value=0  OutDataTypeStr=uint8  SampleTime=0.2
  Memory_controlled : Subsystem
  Reset : Switch  Criteria=u2 ~= 0  Threshold=double(0)  OutDataTypeStr=uint8  SampleTime=0.2  SaturateOnIntegerOverflow=off  InputSameDT=off
  delayMatch : Delay  DelayLength=double(1)  InitialCondition=0  SampleTime=0.2
  delayMatch1 : Delay  DelayLength=double(1)  InitialCondition=0  SampleTime=0.2
  delayMatch2 : Delay  DelayLength=double(1)  InitialCondition=0  SampleTime=0.2
  stateControl : Constant  OutDataTypeStr=boolean  SampleTime=0.2
  y1 : Outport  SampleTime=0.2
  x : Outport  Port=2  SampleTime=0.2
  wires:
  delayMatch/1 -> Reset/1
  Memory_controlled/1(out0) -> FixPt Data Type Duplicate2/1, x/1
  Reset/1 -> Memory_controlled/1(in0), FixPt Data Type Duplicate2/2, y1/1
  delayMatch1/1 -> Memory_controlled/Enable
  u1/1 -> Reset/3, FixPt Data Type Duplicate2/4
  R1/1 -> Reset/2
  delayMatch2/1 -> FixPt Data Type Duplicate2/3
  stateControl/1 -> delayMatch1/1
  Initial Condition/1 -> delayMatch2/1, delayMatch/1

== system gm_robot_fis/MinMax Running Resettable19/Subsystem ==
  note: Reset
  note: Xnew
  note: Xold
  u1 : Inport  OutDataTypeStr=uint8  PortDimensions=1  SampleTime=0.2
  R1 : Inport  Port=2  OutDataTypeStr=uint8  PortDimensions=1  SampleTime=0.2
  FixPt Data Type Duplicate2 : DataTypeDuplicate  DisableCoverage=on  NumInputPorts=4
  Initial Condition : Constant  Value=0  OutDataTypeStr=uint8  SampleTime=0.2
  Memory_controlled : Subsystem
  Reset : Switch  Criteria=u2 ~= 0  Threshold=double(0)  OutDataTypeStr=uint8  SampleTime=0.2  SaturateOnIntegerOverflow=off  InputSameDT=off
  delayMatch : Delay  DelayLength=double(1)  InitialCondition=0  SampleTime=0.2
  delayMatch1 : Delay  DelayLength=double(1)  InitialCondition=0  SampleTime=0.2
  delayMatch2 : Delay  DelayLength=double(1)  InitialCondition=0  SampleTime=0.2
  stateControl : Constant  OutDataTypeStr=boolean  SampleTime=0.2
  y1 : Outport  SampleTime=0.2
  x : Outport  Port=2  SampleTime=0.2
  wires:
  delayMatch/1 -> Reset/1
  Memory_controlled/1(out0) -> FixPt Data Type Duplicate2/1, x/1
  Reset/1 -> Memory_controlled/1(in0), FixPt Data Type Duplicate2/2, y1/1
  delayMatch1/1 -> Memory_controlled/Enable
  u1/1 -> Reset/3, FixPt Data Type Duplicate2/4
  R1/1 -> Reset/2
  delayMatch2/1 -> FixPt Data Type Duplicate2/3
  stateControl/1 -> delayMatch1/1
  Initial Condition/1 -> delayMatch2/1, delayMatch/1

== system gm_robot_fis/MinMax Running Resettable20/Subsystem ==
  note: Reset
  note: Xnew
  note: Xold
  u1 : Inport  OutDataTypeStr=uint8  PortDimensions=1  SampleTime=0.2
  R1 : Inport  Port=2  OutDataTypeStr=uint8  PortDimensions=1  SampleTime=0.2
  FixPt Data Type Duplicate2 : DataTypeDuplicate  DisableCoverage=on  NumInputPorts=4
  Initial Condition : Constant  Value=0  OutDataTypeStr=uint8  SampleTime=0.2
  Memory_controlled : Subsystem
  Reset : Switch  Criteria=u2 ~= 0  Threshold=double(0)  OutDataTypeStr=uint8  SampleTime=0.2  SaturateOnIntegerOverflow=off  InputSameDT=off
  delayMatch : Delay  DelayLength=double(1)  InitialCondition=0  SampleTime=0.2
  delayMatch1 : Delay  DelayLength=double(1)  InitialCondition=0  SampleTime=0.2
  delayMatch2 : Delay  DelayLength=double(1)  InitialCondition=0  SampleTime=0.2
  stateControl : Constant  OutDataTypeStr=boolean  SampleTime=0.2
  y1 : Outport  SampleTime=0.2
  x : Outport  Port=2  SampleTime=0.2
  wires:
  delayMatch/1 -> Reset/1
  Memory_controlled/1(out0) -> FixPt Data Type Duplicate2/1, x/1
  Reset/1 -> Memory_controlled/1(in0), FixPt Data Type Duplicate2/2, y1/1
  delayMatch1/1 -> Memory_controlled/Enable
  u1/1 -> Reset/3, FixPt Data Type Duplicate2/4
  R1/1 -> Reset/2
  delayMatch2/1 -> FixPt Data Type Duplicate2/3
  stateControl/1 -> delayMatch1/1
  Initial Condition/1 -> delayMatch2/1, delayMatch/1

== system gm_robot_fis/MinMax Running Resettable21/Subsystem ==
  note: Reset
  note: Xnew
  note: Xold
  u1 : Inport  OutDataTypeStr=uint8  PortDimensions=1  SampleTime=0.2
  R1 : Inport  Port=2  OutDataTypeStr=uint8  PortDimensions=1  SampleTime=0.2
  FixPt Data Type Duplicate2 : DataTypeDuplicate  DisableCoverage=on  NumInputPorts=4
  Initial Condition : Constant  Value=0  OutDataTypeStr=uint8  SampleTime=0.2
  Memory_controlled : Subsystem
  Reset : Switch  Criteria=u2 ~= 0  Threshold=double(0)  OutDataTypeStr=uint8  SampleTime=0.2  SaturateOnIntegerOverflow=off  InputSameDT=off
  delayMatch : Delay  DelayLength=double(1)  InitialCondition=0  SampleTime=0.2
  delayMatch1 : Delay  DelayLength=double(1)  InitialCondition=0  SampleTime=0.2
  delayMatch2 : Delay  DelayLength=double(1)  InitialCondition=0  SampleTime=0.2
  stateControl : Constant  OutDataTypeStr=boolean  SampleTime=0.2
  y1 : Outport  SampleTime=0.2
  x : Outport  Port=2  SampleTime=0.2
  wires:
  delayMatch/1 -> Reset/1
  Memory_controlled/1(out0) -> FixPt Data Type Duplicate2/1, x/1
  Reset/1 -> Memory_controlled/1(in0), FixPt Data Type Duplicate2/2, y1/1
  delayMatch1/1 -> Memory_controlled/Enable
  u1/1 -> Reset/3, FixPt Data Type Duplicate2/4
  R1/1 -> Reset/2
  delayMatch2/1 -> FixPt Data Type Duplicate2/3
  stateControl/1 -> delayMatch1/1
  Initial Condition/1 -> delayMatch2/1, delayMatch/1

== system gm_robot_fis/MinMax Running Resettable22/Subsystem ==
  note: Reset
  note: Xnew
  note: Xold
  u1 : Inport  OutDataTypeStr=uint8  PortDimensions=1  SampleTime=0.2
  R1 : Inport  Port=2  OutDataTypeStr=uint8  PortDimensions=1  SampleTime=0.2
  FixPt Data Type Duplicate2 : DataTypeDuplicate  DisableCoverage=on  NumInputPorts=4
  Initial Condition : Constant  Value=0  OutDataTypeStr=uint8  SampleTime=0.2
  Memory_controlled : Subsystem
  Reset : Switch  Criteria=u2 ~= 0  Threshold=double(0)  OutDataTypeStr=uint8  SampleTime=0.2  SaturateOnIntegerOverflow=off  InputSameDT=off
  delayMatch : Delay  DelayLength=double(1)  InitialCondition=0  SampleTime=0.2
  delayMatch1 : Delay  DelayLength=double(1)  InitialCondition=0  SampleTime=0.2
  delayMatch2 : Delay  DelayLength=double(1)  InitialCondition=0  SampleTime=0.2
  stateControl : Constant  OutDataTypeStr=boolean  SampleTime=0.2
  y1 : Outport  SampleTime=0.2
  x : Outport  Port=2  SampleTime=0.2
  wires:
  delayMatch/1 -> Reset/1
  Memory_controlled/1(out0) -> FixPt Data Type Duplicate2/1, x/1
  Reset/1 -> Memory_controlled/1(in0), FixPt Data Type Duplicate2/2, y1/1
  delayMatch1/1 -> Memory_controlled/Enable
  u1/1 -> Reset/3, FixPt Data Type Duplicate2/4
  R1/1 -> Reset/2
  delayMatch2/1 -> FixPt Data Type Duplicate2/3
  stateControl/1 -> delayMatch1/1
  Initial Condition/1 -> delayMatch2/1, delayMatch/1

== system gm_robot_fis/MinMax Running Resettable23/Subsystem ==
  note: Reset
  note: Xnew
  note: Xold
  u1 : Inport  OutDataTypeStr=uint8  PortDimensions=1  SampleTime=0.2
  R1 : Inport  Port=2  OutDataTypeStr=uint8  PortDimensions=1  SampleTime=0.2
  FixPt Data Type Duplicate2 : DataTypeDuplicate  DisableCoverage=on  NumInputPorts=4
  Initial Condition : Constant  Value=0  OutDataTypeStr=uint8  SampleTime=0.2
  Memory_controlled : Subsystem
  Reset : Switch  Criteria=u2 ~= 0  Threshold=double(0)  OutDataTypeStr=uint8  SampleTime=0.2  SaturateOnIntegerOverflow=off  InputSameDT=off
  delayMatch : Delay  DelayLength=double(1)  InitialCondition=0  SampleTime=0.2
  delayMatch1 : Delay  DelayLength=double(1)  InitialCondition=0  SampleTime=0.2
  delayMatch2 : Delay  DelayLength=double(1)  InitialCondition=0  SampleTime=0.2
  stateControl : Constant  OutDataTypeStr=boolean  SampleTime=0.2
  y1 : Outport  SampleTime=0.2
  x : Outport  Port=2  SampleTime=0.2
  wires:
  delayMatch/1 -> Reset/1
  Memory_controlled/1(out0) -> FixPt Data Type Duplicate2/1, x/1
  Reset/1 -> Memory_controlled/1(in0), FixPt Data Type Duplicate2/2, y1/1
  delayMatch1/1 -> Memory_controlled/Enable
  u1/1 -> Reset/3, FixPt Data Type Duplicate2/4
  R1/1 -> Reset/2
  delayMatch2/1 -> FixPt Data Type Duplicate2/3
  stateControl/1 -> delayMatch1/1
  Initial Condition/1 -> delayMatch2/1, delayMatch/1

== system gm_robot_fis/MinMax Running Resettable24/Subsystem ==
  note: Reset
  note: Xnew
  note: Xold
  u1 : Inport  OutDataTypeStr=uint8  PortDimensions=1  SampleTime=0.2
  R1 : Inport  Port=2  OutDataTypeStr=uint8  PortDimensions=1  SampleTime=0.2
  FixPt Data Type Duplicate2 : DataTypeDuplicate  DisableCoverage=on  NumInputPorts=4
  Initial Condition : Constant  Value=0  OutDataTypeStr=uint8  SampleTime=0.2
  Memory_controlled : Subsystem
  Reset : Switch  Criteria=u2 ~= 0  Threshold=double(0)  OutDataTypeStr=uint8  SampleTime=0.2  SaturateOnIntegerOverflow=off  InputSameDT=off
  delayMatch : Delay  DelayLength=double(1)  InitialCondition=0  SampleTime=0.2
  delayMatch1 : Delay  DelayLength=double(1)  InitialCondition=0  SampleTime=0.2
  delayMatch2 : Delay  DelayLength=double(1)  InitialCondition=0  SampleTime=0.2
  stateControl : Constant  OutDataTypeStr=boolean  SampleTime=0.2
  y1 : Outport  SampleTime=0.2
  x : Outport  Port=2  SampleTime=0.2
  wires:
  delayMatch/1 -> Reset/1
  Memory_controlled/1(out0) -> FixPt Data Type Duplicate2/1, x/1
  Reset/1 -> Memory_controlled/1(in0), FixPt Data Type Duplicate2/2, y1/1
  delayMatch1/1 -> Memory_controlled/Enable
  u1/1 -> Reset/3, FixPt Data Type Duplicate2/4
  R1/1 -> Reset/2
  delayMatch2/1 -> FixPt Data Type Duplicate2/3
  stateControl/1 -> delayMatch1/1
  Initial Condition/1 -> delayMatch2/1, delayMatch/1

== system gm_robot_fis/MinMax Running Resettable25/Subsystem ==
  note: Reset
  note: Xnew
  note: Xold
  u1 : Inport  OutDataTypeStr=uint8  PortDimensions=1  SampleTime=0.2
  R1 : Inport  Port=2  OutDataTypeStr=uint8  PortDimensions=1  SampleTime=0.2
  FixPt Data Type Duplicate2 : DataTypeDuplicate  DisableCoverage=on  NumInputPorts=4
  Initial Condition : Constant  Value=0  OutDataTypeStr=uint8  SampleTime=0.2
  Memory_controlled : Subsystem
  Reset : Switch  Criteria=u2 ~= 0  Threshold=double(0)  OutDataTypeStr=uint8  SampleTime=0.2  SaturateOnIntegerOverflow=off  InputSameDT=off
  delayMatch : Delay  DelayLength=double(1)  InitialCondition=0  SampleTime=0.2
  delayMatch1 : Delay  DelayLength=double(1)  InitialCondition=0  SampleTime=0.2
  delayMatch2 : Delay  DelayLength=double(1)  InitialCondition=0  SampleTime=0.2
  stateControl : Constant  OutDataTypeStr=boolean  SampleTime=0.2
  y1 : Outport  SampleTime=0.2
  x : Outport  Port=2  SampleTime=0.2
  wires:
  delayMatch/1 -> Reset/1
  Memory_controlled/1(out0) -> FixPt Data Type Duplicate2/1, x/1
  Reset/1 -> Memory_controlled/1(in0), FixPt Data Type Duplicate2/2, y1/1
  delayMatch1/1 -> Memory_controlled/Enable
  u1/1 -> Reset/3, FixPt Data Type Duplicate2/4
  R1/1 -> Reset/2
  delayMatch2/1 -> FixPt Data Type Duplicate2/3
  stateControl/1 -> delayMatch1/1
  Initial Condition/1 -> delayMatch2/1, delayMatch/1

== system gm_robot_fis/MinMax Running Resettable3/Subsystem ==
  note: Reset
  note: Xnew
  note: Xold
  u1 : Inport  OutDataTypeStr=uint8  PortDimensions=1  SampleTime=0.2
  R1 : Inport  Port=2  OutDataTypeStr=uint8  PortDimensions=1  SampleTime=0.2
  FixPt Data Type Duplicate2 : DataTypeDuplicate  DisableCoverage=on  NumInputPorts=4
  Initial Condition : Constant  Value=0  OutDataTypeStr=uint8  SampleTime=0.2
  Memory_controlled : Subsystem
  Reset : Switch  Criteria=u2 ~= 0  Threshold=double(0)  OutDataTypeStr=uint8  SampleTime=0.2  SaturateOnIntegerOverflow=off  InputSameDT=off
  delayMatch : Delay  DelayLength=double(1)  InitialCondition=0  SampleTime=0.2
  delayMatch1 : Delay  DelayLength=double(1)  InitialCondition=0  SampleTime=0.2
  delayMatch2 : Delay  DelayLength=double(1)  InitialCondition=0  SampleTime=0.2
  stateControl : Constant  OutDataTypeStr=boolean  SampleTime=0.2
  y1 : Outport  SampleTime=0.2
  x : Outport  Port=2  SampleTime=0.2
  wires:
  delayMatch/1 -> Reset/1
  Memory_controlled/1(out0) -> FixPt Data Type Duplicate2/1, x/1
  Reset/1 -> Memory_controlled/1(in0), FixPt Data Type Duplicate2/2, y1/1
  delayMatch1/1 -> Memory_controlled/Enable
  u1/1 -> Reset/3, FixPt Data Type Duplicate2/4
  R1/1 -> Reset/2
  delayMatch2/1 -> FixPt Data Type Duplicate2/3
  stateControl/1 -> delayMatch1/1
  Initial Condition/1 -> delayMatch2/1, delayMatch/1
